simulink model "commande_en_effort_avec_boucle_interne_en_position"  (R2024a)
settings: Solver=VariableStepAuto  StartTime=0.0  StopTime=10.0  RelTol=1e-3
values from neighbouring files (symbols this model uses):
  B = diag([3000,3000])    [main.m]
  Fd = [10, 0]'    [main.m]
  K = diag([2500,2500])    [main.m]
  Ke = diag([1E4,0])    [main.m]
  ki = 9e-2    (= 0.09)    [main.m]
  kp = 9e-2    (= 0.09)    [main.m]
  M = diag([500,500])    [main.m]
  Xe = [3,4]'    [main.m]
settings Model: Creator=gabriel  LastModifiedBy=gabriel

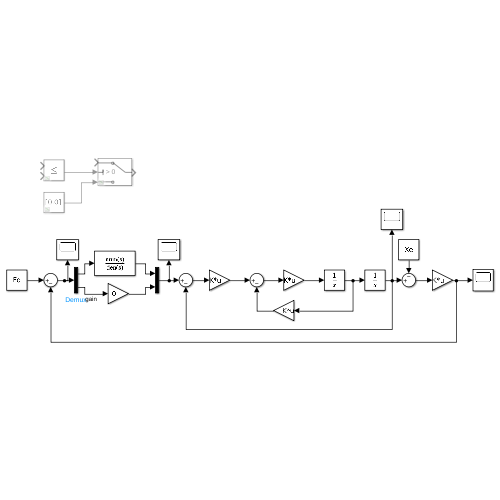
[thumbnail: Simulink's stored preview of the top-level diagram]
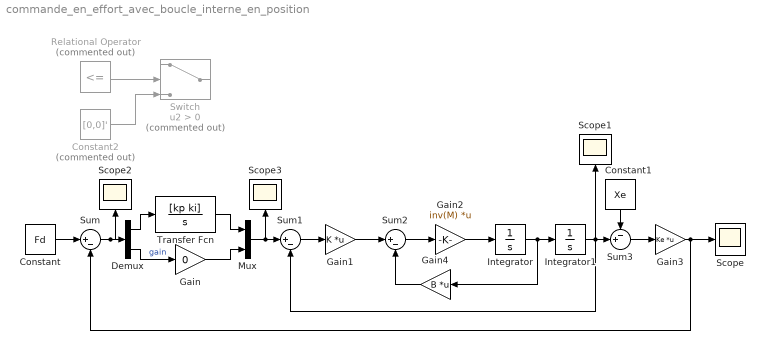
== system commande_en_effort_avec_boucle_interne_en_position ==
  Constant : Constant  Value=Fd
  Constant1 : Constant  Value=Xe
  Constant2 : Constant  Commented=on  Value=[0,0]'
  Demux : Demux  Outputs=2
  Gain : Gain  Gain=0
  Gain1 : Gain  Gain=K  Multiplication=Matrix(K*u)
  Gain2 : Gain  Gain=inv(M)  Multiplication=Matrix(K*u)
  Gain3 : Gain  Gain=Ke  Multiplication=Matrix(K*u)
  Gain4 : Gain  Gain=B  Multiplication=Matrix(K*u)
  Integrator : Integrator
  Integrator1 : Integrator
  Mux : Mux  Inputs=2
  Relational Operator : RelationalOperator  Commented=on  Operator=<=  OutDataTypeStr=boolean  RndMeth=Simplest  InputSameDT=off
  Scope{,1..3} (4 alike) : Scope
  Sum : Sum  Inputs=|+-
  Sum1 : Sum  Inputs=|+-
  Sum2 : Sum  Inputs=|+-
  Sum3 : Sum  Inputs=-+|
  Switch : Switch  Commented=on  Criteria=u2 > Threshold  SaturateOnIntegerOverflow=off  InputSameDT=off
  Transfer Fcn : TransferFcn  Numerator=[kp ki]  Denominator=[1 0]
  wires:
  Constant/1 -> Sum/1
  Gain1/1 -> Sum2/1
  Sum2/1 -> Gain2/1
  Gain2/1 -> Integrator/1
  Integrator/1 -> Gain4/1, Integrator1/1
  Sum3/1 -> Gain3/1
  Gain3/1 -> Sum/2, Scope/1
  Gain4/1 -> Sum2/2
  Integrator1/1 -> Scope1/1, Sum1/2, Sum3/2
  Constant1/1 -> Sum3/1
  Demux/1 -> Transfer Fcn/1
  Transfer Fcn/1 -> Mux/1
  Demux/2 -> Gain/1  "gain"
  Mux/1 -> Scope3/1, Sum1/1
  Sum/1 -> Scope2/1, Demux/1
  Sum1/1 -> Gain1/1
  Relational Operator/1 -> Switch/2
  Constant2/1 -> Switch/3
  Gain/1 -> Mux/2
